simulink model "BLDC_Battery"  (R2024b)
settings: Solver=ode45  StartTime=0.0  StopTime=2.5  RelTol=1e-3  EnableMultiTasking=on
undefined symbols (not defined in the file): Ion, Lithium, sigbuilder_block
libraries: spsDiodeLib x24, spsPermanentMagnetSynchronousMachineLib x2, spsBatteryLib x1, spsSeriesRLCBranchLib x1, spsUniversalBridgeLib x1, sps_lib x1
settings Model: Creator=noname  LastModifiedBy=digvi
settings SolverCC: AlgebraicLoopSolver=TrustRegion
settings DataIOCC: LimitDataPoints=on  SaveFormat=Array  ReturnWorkspaceOutputs=off
settings OptimizationCC: LifeSpan=inf
settings DebuggingCC: UnderspecifiedInitializationDetection=Classic  MergeDetectMultiDrivingBlocksExec=none  SolverPrmCheckMsg=warning  UnconnectedInputMsg=warning  UnconnectedOutputMsg=warning  UnconnectedLineMsg=warning  StateNameClashWarn=warning  SFUnexpectedBacktrackingDiag=warning  SFNoUnconditionalDefaultTransitionDiag=warning  SFExecutionAtInitializationDiag=none  ArithmeticOperatorsInVariantConditions=warning
settings HardwareCC: ProdBitPerPointer=32  ProdBitPerSizeT=32  ProdBitPerPtrDiffT=32  ProdLargestAtomicFloat=None  ProdIntDivRoundTo=Undefined  ProdEndianess=Unspecified  ProdWordSize=32  ProdHWDeviceType=32-bit Generic
settings ModelReferenceCC: EnableRefExpFcnMdlSchedulingChecks=on  PropagateSignalLabelsOutOfModel=off
settings SFSimCC: SimUseLocalCustomCode=off  CustomCodeUndefinedFunction=UseInterfaceOnly
settings RTWCC: RTWUseLocalCustomCode=off  GPUComputeCapability=3.5
settings CodeAppCC: StateflowObjectComments=on
settings GRTTargetCC: TargetLangStandard=C89/C90 (ANSI)
settings ConfigComp: CovMetricSettings=dw  CovSaveCumulativeToWorkspaceVar=on  CovSaveSingleToWorkspaceVar=on  CovExternalEMLEnable=off
settings SimscapeCC: SimscapeNormalizeSystem=off

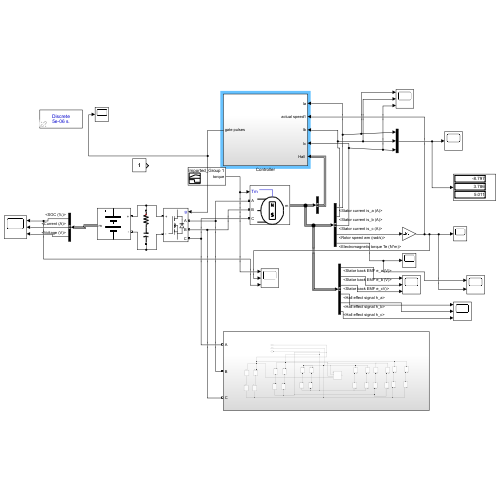
[thumbnail: Simulink's stored preview of the top-level diagram]
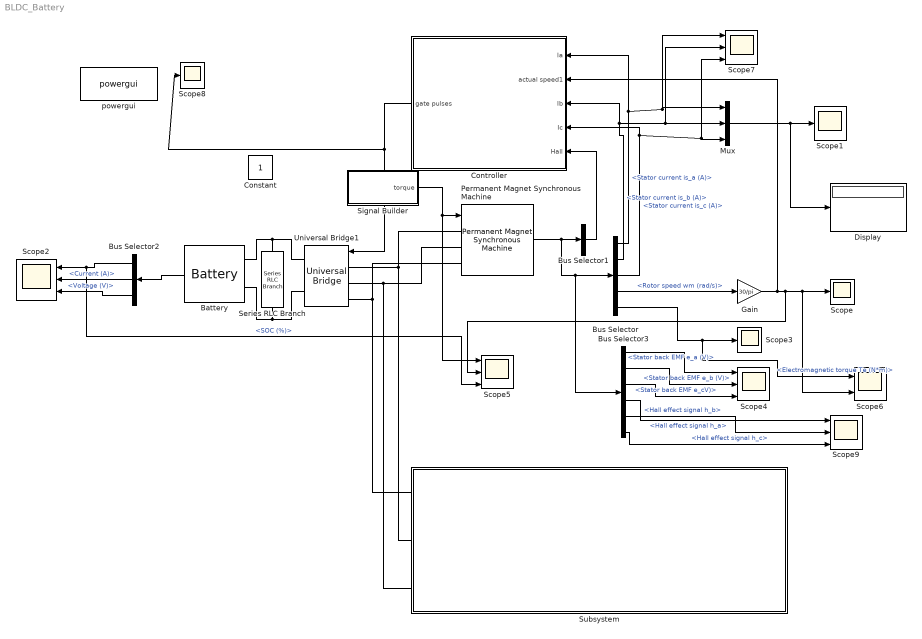
== system BLDC_Battery ==
  Battery : spsBatteryLib/Battery  BatType=Lithium-Ion  NomV=48  NomQ=80  SOC=100  Batt_Tr=3  PresetModel=off  MaxQ=84  MinV=36  FullV=56.818272  Dis_rate=27.82608  R=0.006  Normal_OP=57.87524  expZone=[54.89208 3.144344]
      settings: LibrarySourceBlock=electricdrivelib/Extra Sources/Battery
  Bus Selector : BusSelector  OutputSignals=Stator current is_a (A),Stator current is_b (A),Stator current is_c (A),Rotor speed wm (rad/s),Electromagnetic torque Te (N*m)
  Bus Selector1 : BusSelector  OutputSignals=Hall effect signal h_a,Hall effect signal h_b,Hall effect signal h_c  OutputAsBus=on
  Bus Selector2 : BusSelector  OutputSignals=SOC (%),Current (A),Voltage (V)
  Bus Selector3 : BusSelector  OutputSignals=Stator back EMF e_a (V),Stator back EMF e_b (V),Stator back EMF e_cV),Hall effect signal h_a,Hall effect signal h_b,Hall effect signal h_c
  Constant : Constant
  Controller : Subsystem
  Display : Display
  Gain : Gain  Gain=30/pi
  Mux : Mux  Inputs=3
  Permanent Magnet Synchronous Machine : spsPermanentMagnetSynchronousMachineLib/Permanent Magnet Synchronous Machine  NbPhases=3  FluxDistribution=Trapezoidal  RotorType=Round  MechanicalLoad=Torque Tm  PresetModel=No  ShowDetailedParameters=on  MeasurementBus=off  Resistance=0.0095  Inductance=0.0144e-3  dqInductances=[8.5e-3,8.5e-3]  La=0.000835  MachineConstant=Torque Constant (N.m / A_peak)  Flux=0.0059375  VoltageCst=9.9484  TorqueCst=0.095  Flat=120  Mechanical=[0.00019, 1e-6, 8, 0]  PolePairs=8  InitialConditions=[0,0, 0,0]  InitialConditions5ph=[0 0 0 0 0 0]  RefAngle=90 degrees behind phase A axis (modified Park)  IterativeDiscreteModel=Trapezoidal non iterative  TsBlock=-1  TsPowergui=0
  Scope{,1,3,8} (4 alike) : Scope
  Scope{2,4..5,7,9} (5 alike) : Scope  NumInputPorts=3
  Scope6 : Scope  NumInputPorts=2
  Series RLC Branch : spsSeriesRLCBranchLib/Series RLC Branch  LConnTagsString=__new0  RConnTagsString=__new0  BranchType=RC  Resistance=5  Inductance=1e-3  SetiL0=off  InitialCurrent=0  Capacitance=75e-3  Setx0=off  InitialVoltage=0  Measurements=None
  Signal Builder : Subsystem  Tag=STV Subsys  LoadFcn=sigbuilder_block('load');  StartFcn=sigbuilder_block('start');  StopFcn=sigbuilder_block('stop');  ClipboardFcn=sigbuilder_block('clipboard');  mask(Sigbuilder block){tuvar=[0:10]}
      mask help: Simulink:masks:SigbuilderBlock_MD
      mask init:
      | if ~strcmp(get_param(bdroot(gcbh),'SimulationStatus'),'stopped') tuvar = sigbuilder_block('maskInit'); end
      settings: CopyFcn=sigbuilder_block('copy');  DeleteFcn=sigbuilder_block('delete');  ModelCloseFcn=sigbuilder_block('modelClose');  PreSaveFcn=sigbuilder_block('preSave');  PauseFcn=sigbuilder_block('pause');  ContinueFcn=sigbuilder_block('continue');  NameChangeFcn=sigbuilder_block('namechange');  OpenFcn=sigbuilder_block('open',[437.25 183.75 550.5 395.25 ]);  CloseFcn=sigbuilder_block('close');
      mask Display: plot(0, 0, 100, 100,[2, 2, 32, 32, 2], [68, 8, 8, 68, 68],[32, 2], [38, 38], [32, 19, 2],[53, 60, 44], [32, 17, 17, 2],[16, 16, 31, 31]);txt = getActiveGroup(gcbh);text(2, 100, txt,'verticalAlignment', 'top');
  Subsystem : Subsystem
  Universal Bridge1 : spsUniversalBridgeLib/Universal Bridge  Arms=3  SnubberResistance=1e5  SnubberCapacitance=inf  Device=MOSFET / Diodes  Ron=1e-3  Lon=0  ForwardVoltages="[  0  0  ]"  ForwardVoltage=0  GTOparameters=[ 10e-6 , 20e-6 ]  IGBTparameters=[ 1e-6 , 2e-6 ]  Measurements=None  Measurements_2=None  converterType=Rectifier
  powergui : sps_lib/powergui  Priority=2  SimulationMode=Discrete  SampleTime=5e-6  frequency=60  Iterations=50  frequencyindice=0  Pbase=100e6  ErrMax=1e-4  UnitsV=kV  UnitsW=MW  buscounter=0  FunctionMessages=off  echomessages=off  EnableUseOfTLC=off  CurrentSourceSwitches=off  DisableSnubberDevices=off  DisableRonSwitches=off  DisableVfSwitches=off  DisplayEquations=off  AutomaticDiscreteSolvers=off  SolverType=Tustin  Interpol=off  ExternalGateDelay=off  methode=off  Ts=0  x0status=blocks  SPID=off  SwTol=0  HookPort=off  NonlinearTolerance=1e-4  nMaxIteration=100  ContinueOnMaxIteration=off  RestoreLinks=warning  ResistiveCurrentMeasurement=off  Frange=[0:2:500]  Ylog=off  Xlog=on  ShowGrid=off  save=off  variable=ZData  structure=N  ZoomFFT=off  StartTime=0.0  cycles=1  DisplayStyle=1  fundamental=60  FreqAxis=off  MaxFrequency=1000  frequencyindicesteady=1  RmsSteady=1  display=off
  wires:
  Permanent Magnet Synchronous Machine/1 -> Bus Selector3/1, Bus Selector/1, Bus Selector1/1
  Bus Selector/1 -> Controller/1(Ia), Scope7/1, Mux/1  "<Stator current is_a (A)>"
  Bus Selector/2 -> Scope7/2, Mux/2, Controller/3(Ib)  "<Stator current is_b (A)>"
  Bus Selector/3 -> Scope7/3, Mux/3, Controller/4(Ic)  "<Stator current is_c (A)>"
  Bus Selector/4 -> Gain/1  "<Rotor speed wm (rad/s)>"
  Bus Selector1/1 -> Controller/5("Hall ")
  Gain/1 -> Scope5/2, Scope6/2, Scope/1, Controller/2(actual speed1)
  Controller/1(gate pulses) -> Scope8/1, Universal Bridge1/1
  Battery/1 -> Bus Selector2/1
  Bus Selector2/1 -> Scope5/3, Scope2/1  "<SOC (%)>"
  Bus Selector2/2 -> Scope2/2  "<Current (A)>"
  Bus Selector2/3 -> Scope2/3  "<Voltage (V)>"
  Bus Selector/5 -> Scope6/1, Scope3/1  "<Electromagnetic torque Te (N*m)>"
  Bus Selector3/1 -> Scope4/1  "<Stator back EMF e_a (V)>"
  Bus Selector3/2 -> Scope4/2  "<Stator back EMF e_b (V)>"
  Bus Selector3/3 -> Scope4/3  "<Stator back EMF e_cV)>"
  Mux/1 -> Display/1, Scope1/1
  Signal Builder/1(torque) -> Scope5/1, Permanent Magnet Synchronous Machine/1
  Bus Selector3/4 -> Scope9/1  "<Hall effect signal h_a>"
  Bus Selector3/5 -> Scope9/2  "<Hall effect signal h_b>"
  Bus Selector3/6 -> Scope9/3  "<Hall effect signal h_c>"
  connections:
  Permanent Magnet Synchronous Machine/LConn2 -- Universal Bridge1/LConn2 -- Subsystem/LConn3
  Universal Bridge1/LConn3 -- Permanent Magnet Synchronous Machine/LConn3 -- Subsystem/LConn1
  Series RLC Branch/LConn1 -- Universal Bridge1/RConn1 -- Battery/LConn1
  Series RLC Branch/RConn1 -- Battery/LConn2 -- Universal Bridge1/RConn2
  Universal Bridge1/LConn1 -- Subsystem/LConn2 -- Permanent Magnet Synchronous Machine/LConn1

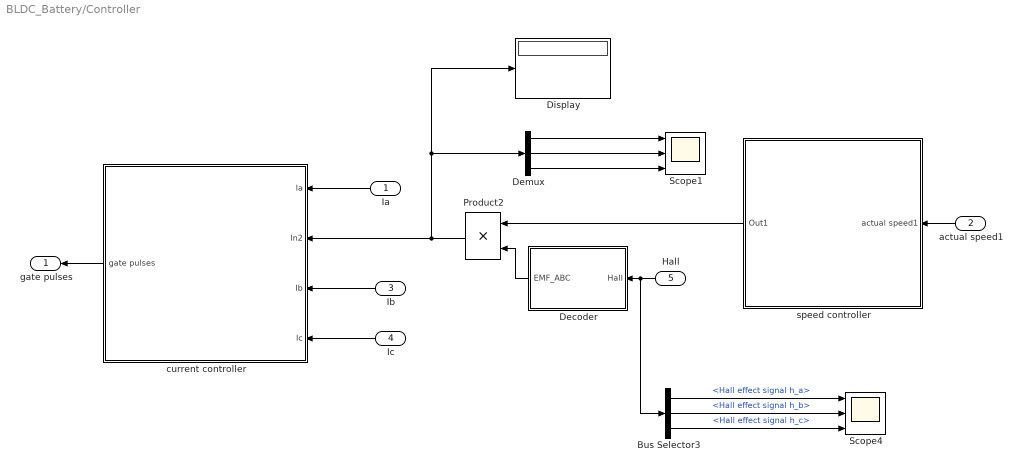
== system BLDC_Battery/Controller ==
  Ia : Inport
  actual speed1 : Inport  Port=2
  Ib : Inport  Port=3
  Ic : Inport  Port=4
  "Hall " : Inport  Port=5
  Bus Selector3 : BusSelector  OutputSignals=Hall effect signal h_a,Hall effect signal h_b,Hall effect signal h_c
  Decoder : Subsystem
  Demux : Demux  Outputs=3
  Display : Display
  Product2 : Product  SaturateOnIntegerOverflow=on  OutDataTypeStr=Inherit: Same as first input
  Scope1 : Scope  NumInputPorts=3
  Scope4 : Scope  NumInputPorts=3
  current controller : Subsystem
  speed controller : Subsystem
  gate pulses : Outport  VectorParamsAs1DForOutWhenUnconnected=off
  wires:
  "Hall "/1 -> Bus Selector3/1, Decoder/1(Hall)
  current controller/1(gate pulses) -> gate pulses/1
  Ic/1 -> current controller/4(Ic)
  Ib/1 -> current controller/3(Ib)
  Ia/1 -> current controller/1(Ia)
  Product2/1 -> Demux/1, Display/1, current controller/2(In2)
  actual speed1/1 -> speed controller/1(actual speed1)
  speed controller/1(Out1) -> Product2/1
  Bus Selector3/1 -> Scope4/1  "<Hall effect signal h_a>"
  Bus Selector3/2 -> Scope4/2  "<Hall effect signal h_b>"
  Bus Selector3/3 -> Scope4/3  "<Hall effect signal h_c>"
  Demux/1 -> Scope1/1
  Demux/2 -> Scope1/2
  Demux/3 -> Scope1/3
  Decoder/1(EMF_ABC) -> Product2/2

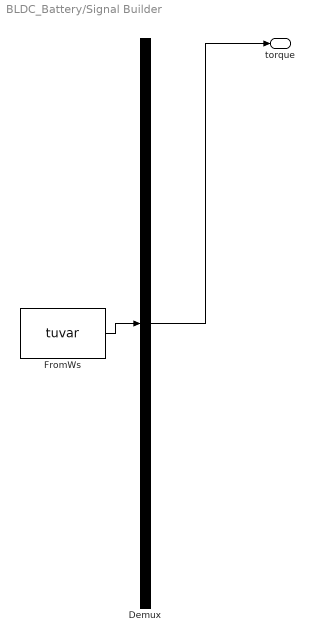
== system BLDC_Battery/Signal Builder ==
  Demux : Demux  Tag=STV Demux  Outputs=1
      settings: DisplayOption=none
  FromWs : FromWorkspace  Tag=STV FromWs  VariableName=tuvar
      SigBuilderData=|
      | common.afterFinalStr = 'Extrapolate'
      | common.sampleTime = 0
      | dataSet.timeRange = [0 2.5]
      | dataSet.name = 'Imported_Group 1'
      | sbobj.Name = 'Signal Builder'
      | sbobj.Groups.Name = 'Imported_Group 1'
      | sbobj.Groups.Signals.Name = 'torque'
      | sbobj.Groups.Signals.XData = [0 0.05 0.05 0.5 0.5 0.75 0.75 1.25 1.25 1.65 1.65 2.05 2.05 2.35 2.35 2.5]
      | sbobj.Groups.Signals.YData = [0 0 5 5 4 4 -3 -3 1.5 1.5 5 5 4 4 -1 -1]
      | sbobj.Groups.TimeRange = [0 2.5]
  torque : Outport  VectorParamsAs1DForOutWhenUnconnected=off
  wires:
  Demux/1 -> torque/1
  FromWs/1 -> Demux/1

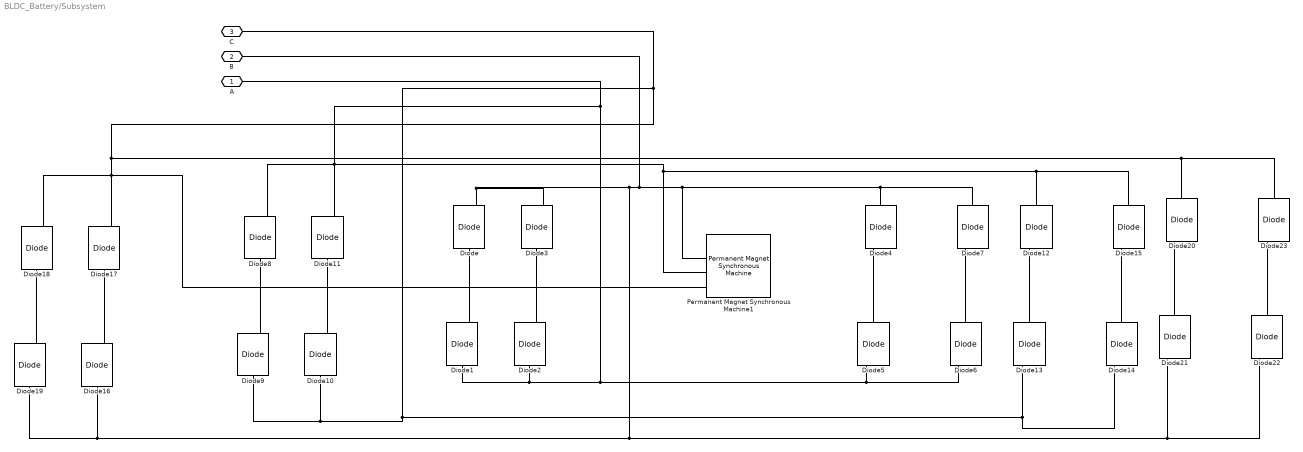
== system BLDC_Battery/Subsystem ==
  Diode{,1..23} (24 alike) : spsDiodeLib/Diode  Ron=0.001  Lon=0  Vf=0.8  IC=0  UseSnubber=0  Rs=500  Cs=250e-9  Measurements=on
  Permanent Magnet Synchronous Machine1 : spsPermanentMagnetSynchronousMachineLib/Permanent Magnet Synchronous Machine  NbPhases=3  FluxDistribution=Trapezoidal  RotorType=Round  MechanicalLoad=Torque Tm  PresetModel=No  ShowDetailedParameters=on  MeasurementBus=off  Resistance=0.0095  Inductance=0.0144e-3  dqInductances=[8.5e-3,8.5e-3]  La=0.000835  MachineConstant=Torque Constant (N.m / A_peak)  Flux=0.0059375  VoltageCst=9.9484  TorqueCst=0.095  Flat=120  Mechanical=[0.00019, 1e-6, 8, 0]  PolePairs=8  InitialConditions=[0,0, 0,0]  InitialConditions5ph=[0 0 0 0 0 0]  RefAngle=90 degrees behind phase A axis (modified Park)  IterativeDiscreteModel=Trapezoidal non iterative  TsBlock=-1  TsPowergui=0
  A : PMIOPort  Side=Left
  B : PMIOPort  Port=2  Side=Left
  C : PMIOPort  Port=3  Side=Left
  connections:
  Diode8/RConn1 -- Diode12/LConn1 -- Diode15/LConn1 -- Permanent Magnet Synchronous Machine1/LConn2 -- Diode11/RConn1 -- A/RConn1 -- Diode2/LConn1 -- Diode1/LConn1 -- Diode6/RConn1 -- Diode5/RConn1
  Diode7/LConn1 -- Diode4/LConn1 -- Permanent Magnet Synchronous Machine1/LConn1 -- Diode22/RConn1 -- Diode21/RConn1 -- Diode16/LConn1 -- Diode19/LConn1 -- Diode/RConn1 -- Diode3/RConn1 -- B/RConn1
  Permanent Magnet Synchronous Machine1/LConn3 -- Diode17/RConn1 -- Diode18/RConn1 -- C/RConn1 -- Diode10/LConn1 -- Diode9/LConn1 -- Diode14/RConn1 -- Diode13/RConn1 -- Diode23/LConn1 -- Diode20/LConn1
  Diode5/LConn1 -- Diode4/RConn1
  Diode2/RConn1 -- Diode3/LConn1
  Diode13/LConn1 -- Diode12/RConn1
  Diode21/LConn1 -- Diode20/RConn1
  Diode1/RConn1 -- Diode/LConn1
  Diode9/RConn1 -- Diode8/LConn1
  Diode15/RConn1 -- Diode14/LConn1
  Diode7/RConn1 -- Diode6/LConn1
  Diode10/RConn1 -- Diode11/LConn1
  Diode23/RConn1 -- Diode22/LConn1
  Diode16/RConn1 -- Diode17/LConn1
  Diode19/RConn1 -- Diode18/LConn1

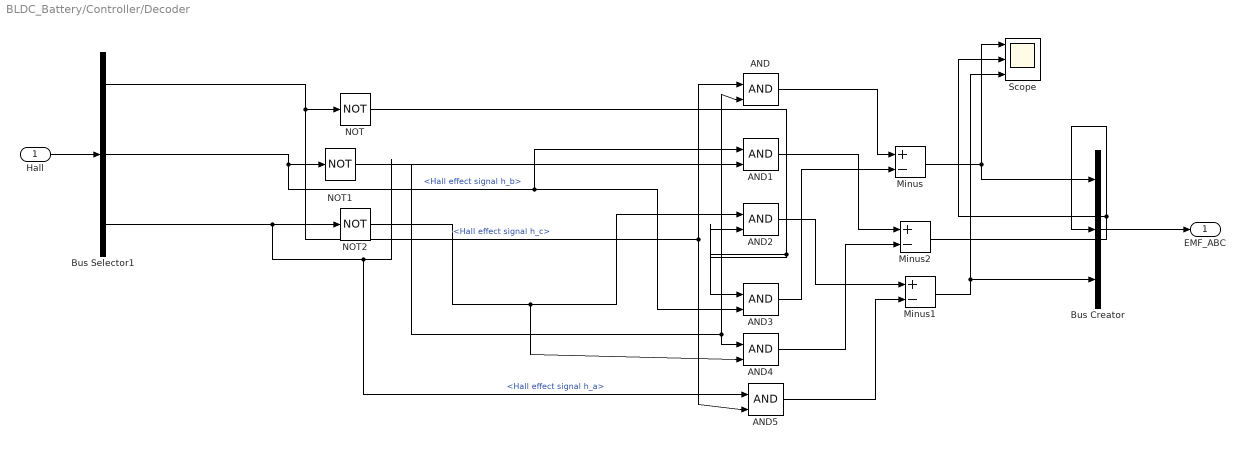
== system BLDC_Battery/Controller/Decoder ==
  Hall : Inport
  AND{,1..5} (6 alike) : Logic  IconShape=distinctive  AllPortsSameDT=off  OutDataTypeStr=boolean
  Bus Creator : BusCreator  Inputs=3
  Bus Selector1 : BusSelector  OutputSignals=Hall effect signal h_c,Hall effect signal h_b,Hall effect signal h_a
  Minus : Sum  Inputs=+-
  Minus1 : Sum  Inputs=+-
  Minus2 : Sum  Inputs=+-
  NOT : Logic  Operator=NOT  IconShape=distinctive  AllPortsSameDT=off  OutDataTypeStr=boolean
  NOT1 : Logic  Operator=NOT  IconShape=distinctive  AllPortsSameDT=off  OutDataTypeStr=boolean
  NOT2 : Logic  Operator=NOT  IconShape=distinctive  AllPortsSameDT=off  OutDataTypeStr=boolean
  Scope : Scope  NumInputPorts=3
  EMF_ABC : Outport
  wires:
  Hall/1 -> Bus Selector1/1
  AND5/1 -> Minus1/2
  NOT/1 -> AND3/1, AND2/2
  AND3/1 -> Minus/2
  Bus Selector1/3 -> AND5/1, AND1/2, NOT2/1  "<Hall effect signal h_a>"
  AND4/1 -> Minus2/2
  AND2/1 -> Minus1/1
  Minus/1 -> Bus Creator/1, Scope/1
  AND/1 -> Minus/1
  NOT1/1 -> AND4/1, AND/2
  AND1/1 -> Minus2/1
  Minus1/1 -> Bus Creator/3, Scope/3
  Minus2/1 -> Scope/2, Bus Creator/2
  Bus Selector1/1 -> AND5/2, AND/1, NOT/1  "<Hall effect signal h_c>"
  NOT2/1 -> AND4/2, AND2/1
  Bus Selector1/2 -> AND3/2, AND1/1, NOT1/1  "<Hall effect signal h_b>"
  Bus Creator/1 -> EMF_ABC/1

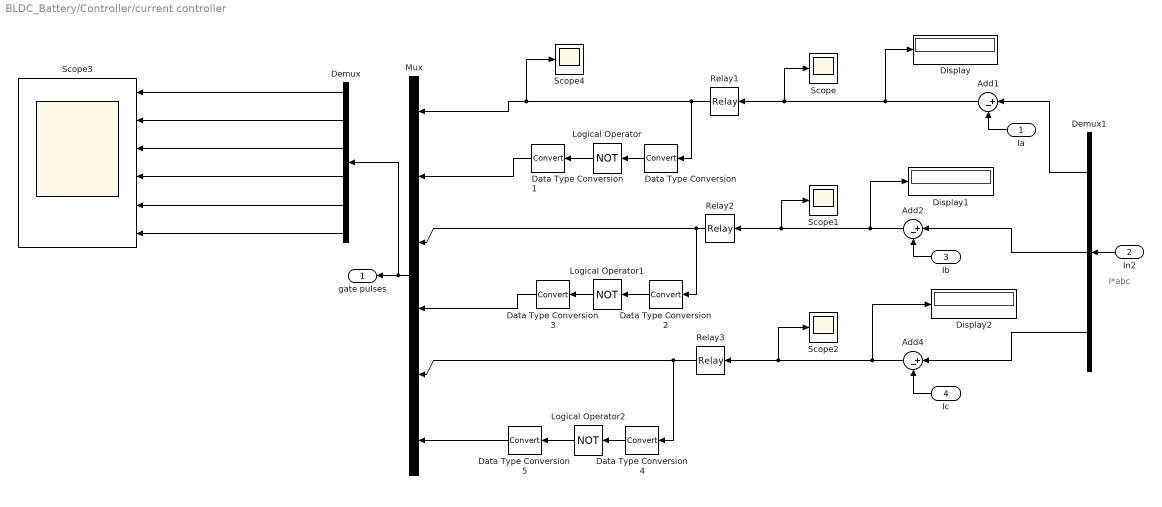
== system BLDC_Battery/Controller/current controller ==
  note: I*abc
  Ia : Inport
  In2 : Inport  Port=2
  Ib : Inport  Port=3
  Ic : Inport  Port=4
  Add1 : Sum  Inputs=|+-
  Add2 : Sum  Inputs=|+-
  Add4 : Sum  Inputs=|+-
  Data Type Conversion{,1..5} (6 alike) : DataTypeConversion
  Demux : Demux  Outputs=6
  Demux1 : Demux  Outputs=3
      settings: DisplayOption=none
  Display : Display
  Display1 : Display
  Display2 : Display
  Logical Operator : Logic  Operator=NOT  AllPortsSameDT=off  OutDataTypeStr=boolean
  Logical Operator1 : Logic  Operator=NOT  AllPortsSameDT=off  OutDataTypeStr=boolean
  Logical Operator2 : Logic  Operator=NOT  AllPortsSameDT=off  OutDataTypeStr=boolean
  Mux : Mux  Inputs=6
  Relay1 : Relay  OnSwitchValue=5  OffSwitchValue=-5
  Relay2 : Relay  OnSwitchValue=5  OffSwitchValue=-5
  Relay3 : Relay  OnSwitchValue=5  OffSwitchValue=-5
  Scope{,1..2,4} (4 alike) : Scope
  Scope3 : Scope  NumInputPorts=6
  gate pulses : Outport  VectorParamsAs1DForOutWhenUnconnected=off
  wires:
  Relay1/1 -> Scope4/1, Mux/1, Data Type Conversion/1
  Relay2/1 -> Mux/3, Data Type Conversion2/1
  Relay3/1 -> Mux/5, Data Type Conversion4/1
  Ib/1 -> Add2/2
  Mux/1 -> Demux/1, gate pulses/1
  Ic/1 -> Add4/2
  Add4/1 -> Display2/1, Scope2/1, Relay3/1
  Add2/1 -> Display1/1, Scope1/1, Relay2/1
  Add1/1 -> Display/1, Scope/1, Relay1/1
  Data Type Conversion/1 -> Logical Operator/1
  Logical Operator/1 -> Data Type Conversion1/1
  Data Type Conversion1/1 -> Mux/2
  Logical Operator1/1 -> Data Type Conversion3/1
  Data Type Conversion3/1 -> Mux/4
  Data Type Conversion2/1 -> Logical Operator1/1
  Data Type Conversion5/1 -> Mux/6
  Logical Operator2/1 -> Data Type Conversion5/1
  Data Type Conversion4/1 -> Logical Operator2/1
  Demux1/2 -> Add2/1
  Demux1/3 -> Add4/1
  In2/1 -> Demux1/1
  Ia/1 -> Add1/2
  Demux1/1 -> Add1/1
  Demux/1 -> Scope3/1
  Demux/2 -> Scope3/2
  Demux/3 -> Scope3/3
  Demux/4 -> Scope3/4
  Demux/5 -> Scope3/5
  Demux/6 -> Scope3/6

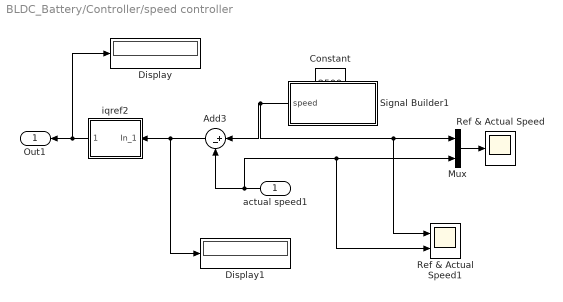
== system BLDC_Battery/Controller/speed controller ==
  actual speed1 : Inport
  Add3 : Sum  Inputs=|+-
  Constant : Constant  Value=2500
  Display : Display
  Display1 : Display
  Mux : Mux  Inputs=2
  Ref & Actual Speed : Scope
  Ref & Actual Speed1 : Scope  NumInputPorts=2
  Signal Builder1 : Subsystem  Tag=STV Subsys  LoadFcn=sigbuilder_block('load');  StartFcn=sigbuilder_block('start');  StopFcn=sigbuilder_block('stop');  ClipboardFcn=sigbuilder_block('clipboard');  mask(Sigbuilder block){tuvar=[0:10]}
      mask help: Simulink:masks:SigbuilderBlock_MD
      mask init:
      | if ~strcmp(get_param(bdroot(gcbh),'SimulationStatus'),'stopped') tuvar = sigbuilder_block('maskInit'); end
      settings: CopyFcn=sigbuilder_block('copy');  DeleteFcn=sigbuilder_block('delete');  ModelCloseFcn=sigbuilder_block('modelClose');  PreSaveFcn=sigbuilder_block('preSave');  PauseFcn=sigbuilder_block('pause');  ContinueFcn=sigbuilder_block('continue');  NameChangeFcn=sigbuilder_block('namechange');  OpenFcn=sigbuilder_block('open',[6.75 6.75 1138.5 568.5 ]);  CloseFcn=sigbuilder_block('close');
      mask Display: plot(0, 0, 100, 100,[2, 2, 32, 32, 2], [68, 8, 8, 68, 68],[32, 2], [38, 38], [32, 19, 2],[53, 60, 44], [32, 17, 17, 2],[16, 16, 31, 31]);txt = getActiveGroup(gcbh);text(2, 100, txt,'verticalAlignment', 'top');
  iqref2 : Subsystem  mask(PI Controller){I=2.8, P=5, sat=[-inf, inf]}
      mask prompts: I "Integral"; P "Proportional:"; sat "Minimum and maximum outputs:"
      mask init:
      | min=sat(1);max=sat(2);
      mask Display: disp('PI')
  Out1 : Outport  VectorParamsAs1DForOutWhenUnconnected=off
  wires:
  Add3/1 -> Display1/1, iqref2/1(In_1)
  iqref2/1(Out_1) -> Display/1, Out1/1
  Mux/1 -> Ref & Actual Speed/1
  actual speed1/1 -> Ref & Actual Speed1/2, Mux/2, Add3/2
  Signal Builder1/1(speed) -> Ref & Actual Speed1/1, Mux/1, Add3/1

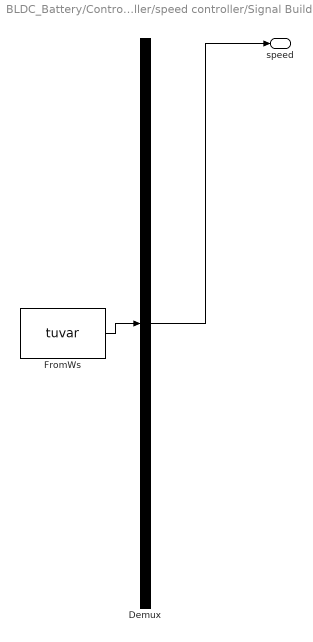
== system BLDC_Battery/Controller/speed controller/Signal Builder1 ==
  Demux : Demux  Tag=STV Demux  Outputs=1
      settings: DisplayOption=none
  FromWs : FromWorkspace  Tag=STV FromWs  VariableName=tuvar
      SigBuilderData=|
      | common.afterFinalStr = 'Extrapolate'
      | common.sampleTime = 0
      | dataSet.timeRange = [0 2.5]
      | dataSet.name = 'Imported_Group 1'
      | sbobj.Name = 'Signal Builder'
      | sbobj.Groups.Name = 'Imported_Group 1'
      | sbobj.Groups.Signals.Name = 'speed'
      | sbobj.Groups.Signals.XData = [0 0.05 0.5 0.75 1.25 1.65 2.05 2.35 2.5]
      | sbobj.Groups.Signals.YData = [0 0 2500 2500 1000 1000 2000 2000 1000]
      | sbobj.Groups.TimeRange = [0 2.5]
  speed : Outport  VectorParamsAs1DForOutWhenUnconnected=off
  wires:
  Demux/1 -> speed/1
  FromWs/1 -> Demux/1

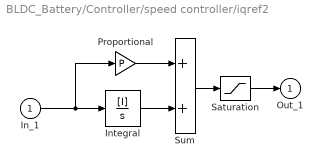
== system BLDC_Battery/Controller/speed controller/iqref2 ==
  In_1 : Inport
  Integral : TransferFcn  Numerator=[I]  Denominator=[1 0]
  Proportional : Gain  Gain=P  SaturateOnIntegerOverflow=on  OutDataTypeStr=Inherit: Same as input  ParamDataTypeStr=Inherit: Same as input
  Saturation : Saturate  UpperLimit=max  LowerLimit=min
  Sum : Sum  InputSameDT=on  SaturateOnIntegerOverflow=on  OutDataTypeStr=Inherit: Same as first input
  Out_1 : Outport  InitialOutput=0  VectorParamsAs1DForOutWhenUnconnected=off
  wires:
  Integral/1 -> Sum/2
  In_1/1 -> Integral/1, Proportional/1
  Proportional/1 -> Sum/1
  Sum/1 -> Saturation/1
  Saturation/1 -> Out_1/1
